simulink model "prob_2"  (R2020b)
settings: Solver=VariableStepAuto  StartTime=0.0  StopTime=10.0  RelTol=1e-3
model workspace (MAT data in the model file):
  K1 = 80000
  K2 = 500000
  M1 = 2500
  M2 = 320
  b = 350
settings Model: Creator=Lakshmi  LastModifiedBy=Lakshmi

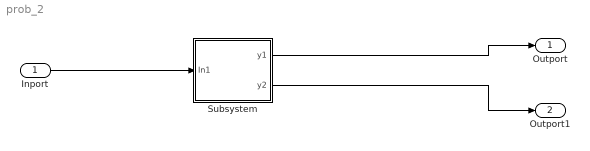
== system prob_2 ==
  Inport : Inport
  Subsystem : Subsystem
  Outport : Outport
  Outport1 : Outport  Port=2
  wires:
  Inport/1 -> Subsystem/1(In1)
  Subsystem/1(y1) -> Outport/1
  Subsystem/2(y2) -> Outport1/1

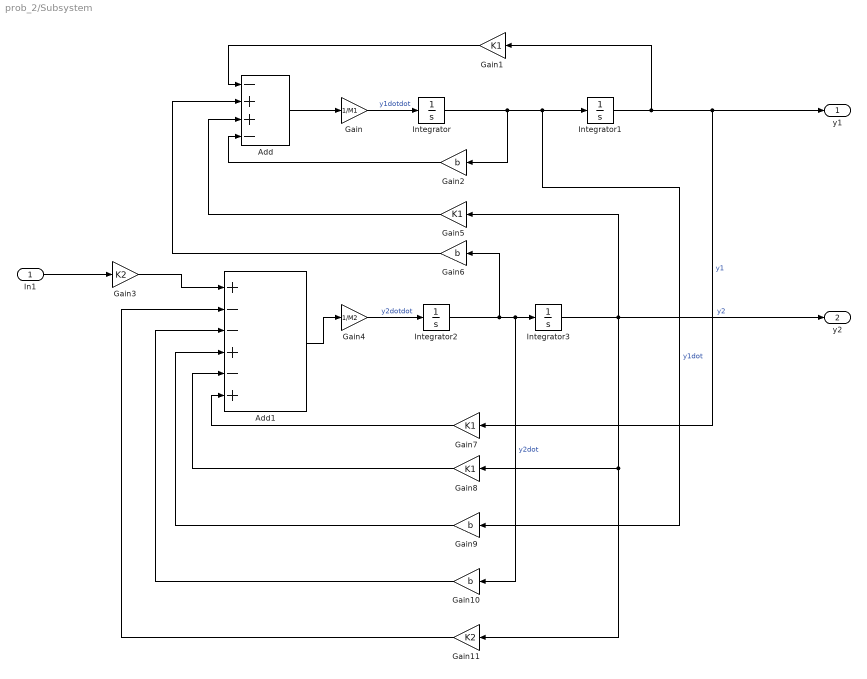
== system prob_2/Subsystem ==
  In1 : Inport
  Add : Sum  Inputs=-++-
  Add1 : Sum  Inputs=+--+-+
  Gain : Gain  Gain=1/M1
  Gain{1,5,7..8} (4 alike) : Gain  Gain=K1
  Gain{2,6,9..10} (4 alike) : Gain  Gain=b
  Gain11 : Gain  Gain=K2
  Gain3 : Gain  Gain=K2
  Gain4 : Gain  Gain=1/M2
  Integrator{,1..3} (4 alike) : Integrator
  y1 : Outport
  y2 : Outport  Port=2
  wires:
  Gain3/1 -> Add1/1
  Gain11/1 -> Add1/2
  Gain1/1 -> Add/1
  Add/1 -> Gain/1
  Integrator3/1 -> y2/1, Gain11/1, Gain8/1, Gain5/1  "y2"
  Gain/1 -> Integrator/1  "y1dotdot"
  Integrator/1 -> Gain2/1, Gain9/1, Integrator1/1  "y1dot"
  Gain7/1 -> Add1/6
  Integrator1/1 -> Gain1/1, y1/1, Gain7/1  "y1"
  Integrator2/1 -> Gain6/1, Gain10/1, Integrator3/1  "y2dot"
  Gain2/1 -> Add/4
  Gain8/1 -> Add1/5
  Gain10/1 -> Add1/3
  Add1/1 -> Gain4/1
  Gain4/1 -> Integrator2/1  "y2dotdot"
  In1/1 -> Gain3/1
  Gain9/1 -> Add1/4
  Gain6/1 -> Add/2
  Gain5/1 -> Add/3
